simulink model "AWident_2015"  (Simulink 8.6)
settings: Solver=ode45  StartTime=0.0  StopTime=tend  MaxStep=0.01  RelTol=1e-3
InitFcn:
  | N = 1001;
  | Tp = 0.5;
  | sigma2v = 0.001;
  | tend = 500;
libraries: simulink x1
settings Model: Creator=mgmil  LastModifiedBy=mgmil
settings OptimizationCC: ExpressionDepthLimit=128  InitFltsAndDblsToZero=on
settings DebuggingCC: SaveWithParameterizedLinksMsg=none  SignalResolutionControl=TryResolveAllWithWarning  MultiTaskDSMMsg=warning  MultiTaskCondExecSysMsg=none  FcnCallInpInsideContextMsg=EnableAllAsWarning  AllowSymbolicDim=on  StateNameClashWarn=none
settings SFSimCC: SimUseLocalCustomCode=on
settings RTWCC: RTWUseLocalCustomCode=on
settings GRTTargetCC: TargetFcnLib=ansi_tfl_tmw.mat  GeneratePreprocessorConditionals=Use local settings
settings ConfigComp: CovExternalEMLEnable=on

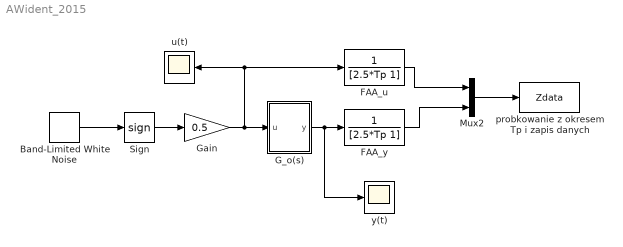
== system AWident_2015 ==
  Band-Limited White Noise : simulink/Sources/Band-Limited White Noise  Cov=[0.5]*Tp  Ts=Tp  seed=[23341]
  FAA_u : TransferFcn  Denominator=[2.5*Tp 1]
  FAA_y : TransferFcn  Denominator=[2.5*Tp 1]
  G_o(s) : Subsystem
  Gain : Gain  Gain=0.5
  Mux2 : Mux  Inputs=2
  Sign : Signum  ZeroCross=off
  probkowanie z okresem Tp i zapis danych : ToWorkspace  VariableName=Zdata  SampleTime=Tp
  u(t) : Scope
  y(t) : Scope
  wires:
  Band-Limited White Noise/1 -> Sign/1
  Sign/1 -> Gain/1
  Gain/1 -> G_o(s)/1(u), FAA_u/1, u(t)/1
  G_o(s)/1(y) -> FAA_y/1, y(t)/1
  FAA_u/1 -> Mux2/1
  FAA_y/1 -> Mux2/2
  Mux2/1 -> probkowanie z okresem Tp i zapis danych/1

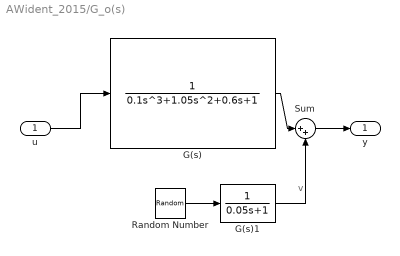
== system AWident_2015/G_o(s) ==
  note: v
  u : Inport
  G(s) : TransferFcn  Denominator=[0.1 1.05 0.6 1]
  G(s)1 : TransferFcn  Denominator=[0.05 1]
  Random Number : RandomNumber  Variance=sigma2v  Seed=159  SampleTime=Tp*0.1
  Sum : Sum  Inputs=|++
  y : Outport
  wires:
  G(s)/1 -> Sum/1
  u/1 -> G(s)/1
  Sum/1 -> y/1
  G(s)1/1 -> Sum/2
  Random Number/1 -> G(s)1/1
